simulink model "constant_blocks"  (R2020b)
settings: Solver=VariableStepAuto  StartTime=0.0  StopTime=10.0  RelTol=1e-3
settings Model: Creator=Lenovo  LastModifiedBy=Lenovo

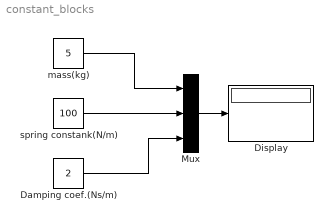
== system constant_blocks ==
  Damping coef.(Ns/m) : Constant  Value=2
  Display : Display
  Mux : Mux  Inputs=3
  mass(kg) : Constant  Value=5
  spring constank(N/m) : Constant  Value=100
  wires:
  spring constank(N/m)/1 -> Mux/2
  mass(kg)/1 -> Mux/1
  Damping coef.(Ns/m)/1 -> Mux/3
  Mux/1 -> Display/1
